simulink model "HeliDraft_06_02_2025_13_24pm"  (R2024b)
settings: Solver=VariableStepAuto  StartTime=0.0  StopTime=10.0  RelTol=1e-3
undefined symbols (not defined in the file or in its folder): AngVel, AngVeltr, Earth, MTOW, WGS84
libraries: aerolibatmos2 x2, aerolibanimutils x2, aerolibfltsims x2, aerolibtransform2 x1, shared6dof x1
settings Model: Creator=stand-alone1  LastModifiedBy=stand-alone1

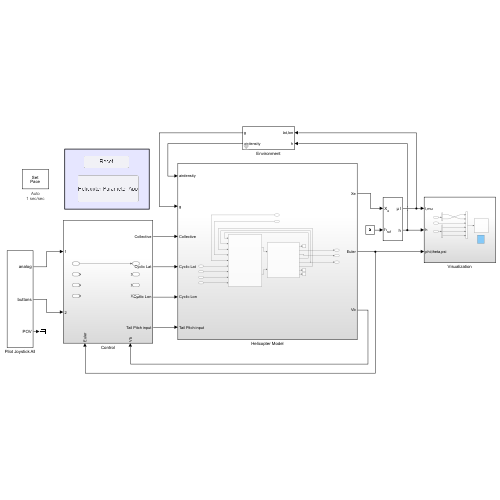
[thumbnail: Simulink's stored preview of the top-level diagram]
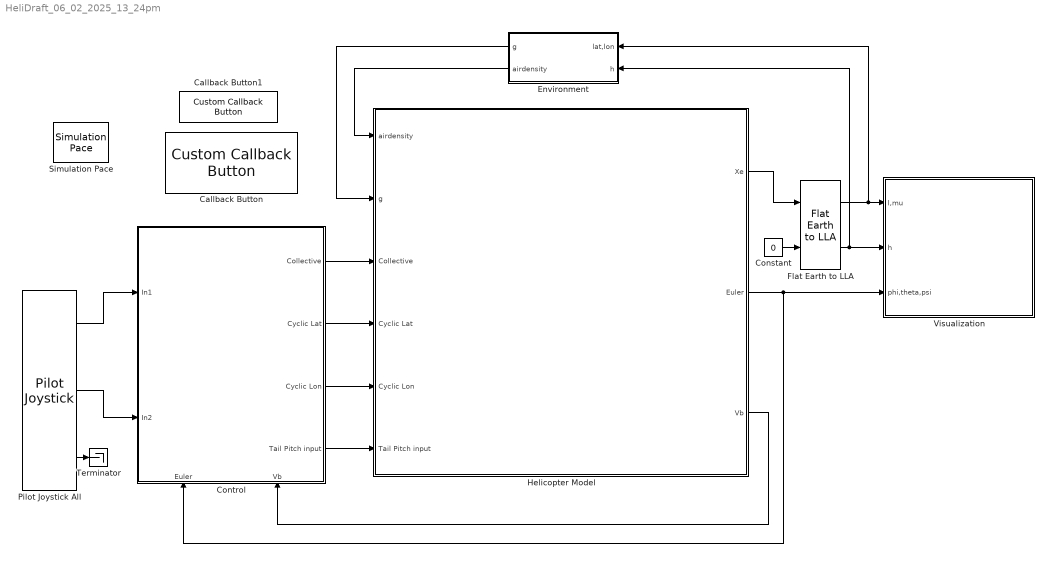
== system HeliDraft_06_02_2025_13_24pm ==
  Callback Button : CustomCallbackButton  Configuration="{\"components\":[{\"name\":\"BackgroundImageComponent\",\"settings\":{\"image\":{\"size\":[0,0],\"src\":\"default\",\"srcOrientation\":\"Right\"},\"position\":[0,0,1,1]}},{\"name\":\"ButtonStateComponent\",\"settings\":{\"buttonType\":\"momentary\",\"clickFcn\":\"run(\\\"HelicopterParameterEstimation.mlapp\\\");\",\"onValue\":1,\"position\":[0,0,1,1],\"pressDelay\":\"500\",\"pressFcn\":\"\",\"repeatInterval\":\"0\",\"states\":[{\"horizontalAlignment\":\"center\",\"image\":{\"position\":[0,0,1,1],\"size\":[1,1],\"src\":\"default\",\"srcOrientation\":\"Right\"},\"label\":{\"color\":[0.01176470588,0.01176470588,0.01176470588,1],\"icon\":{\"size\":[0,0],\"src\":\"default\",\"srcOrientation\":\"Right\"},\"iconOffset\":0,\"iconPlacement\":\"left\",\"opacity\":1,\"show\":true,\"text\":{\"content\":\"Helicopter Parameter App\",\"font\":\"Helvetica\"}},\"labelOffset\":[0,0],\"verticalAlignment\":\"middle\"},{\"horizontalAlignment\":\"center\",\"image\":{\"position\":[0,0,1,1],\"size\":[1,1],\"src\":\"default\",\"srcOrientation\":\"Right\"},\"label\":{\"color\":[0.01176470588,0.01176470588,0.01176470588,1],\"icon\":{\"size\":[0,0],\"src\":\"default\",\"srcOrientation\":\"Right\"},\"iconOffset\":0,\"iconPlacement\":\"left\",\"opacity\":1,\"show\":true,\"text\":{\"content\":\"Helicopter Parameter App\",\"font\":\"Helvetica\"}},\"labelOffset\":[0,0],\"verticalAlignment\":\"middle\"},{\"horizontalAlignment\":\"center\",\"image\":{\"position\":[0,0,1,1],\"size\":[1,1],\"src\":\"default\",\"srcOrientation\":\"Right\"},\"label\":{\"color\":[0.01176470588,0.01176470588,0.01176470588,1],\"icon\":{\"size\":[0,0],\"src\":\"default\",\"srcOrientation\":\"Right\"},\"iconOffset\":0,\"iconPlacement\":\"left\",\"opacity\":1,\"show\":true,\"text\":{\"content\":\"Helicopter Parameter App\",\"font\":\"Helvetica\"}},\"labelOffset\":[0,0],\"verticalAlignment\":\"middle\"},{\"horizontalAlignment\":\"center\",\"image\":{\"position\":[0,0,1,1],\"size\":[1,1],\"src\":\"default\",\"srcOrientation\":\"Right\"},\"label\":{\"color\":[0.01176470588,0.01176470588,0.01176470588,1],\"icon\":{\"size\":[0,0],\"src\":\"default\",\"srcOrientation\":\"Right\"},\"iconOffset\":0,\"iconPlacement\":\"left\",\"opacity\":1,\"show\":true,\"text\":{\"content\":\"Helicopter Parameter App\",\"font\":\"Helvetica\"}},\"labelOffset\":[0,0],\"verticalAlignment\":\"middle\"}]}},{\"name\":\"ForegroundImageComponent\",\"settings\":{\"image\":{\"size\":[0,0],\"src\":\"default\",\"srcOrientation\":\"Right\"},\"isForeground\":1,\"position\":[0,0,1,1]}}],\"settings\":{\"BindingType\":\"standalone\",\"backgroundColor\":[244,244,244,1],\"backgroundOffset\":0.2,\"backgroundOpacity\":1,\"fixedAspectRatio\":\"off\",\"foregroundColor\":[0.01176470588,0.01176470588,0.01176470588,1],\"migratedFromLegacy\":true,\"useBackgroundColor\":true,\"variant\":\"callback\",\"version\":\"R2023a\"},\"type\":\"Button\"}"  CustomBackgroundColor="{\"color\":[0.9568627451,0.9568627451,0.9568627451],\"show\":true}"
  Callback Button1 : CustomCallbackButton  Configuration="{\"components\":[{\"name\":\"BackgroundImageComponent\",\"settings\":{\"image\":{\"size\":[0,0],\"src\":\"default\",\"srcOrientation\":\"Right\"},\"position\":[0,0,1,1]}},{\"name\":\"ButtonStateComponent\",\"settings\":{\"buttonType\":\"momentary\",\"clickFcn\":\"clc; clear; close all;\",\"onValue\":1,\"position\":[0,0,1,1],\"pressDelay\":\"500\",\"pressFcn\":\"\",\"repeatInterval\":\"0\",\"states\":[{\"horizontalAlignment\":\"center\",\"image\":{\"position\":[0,0,1,1],\"size\":[1,1],\"src\":\"default\",\"srcOrientation\":\"Right\"},\"label\":{\"color\":[0.01176470588,0.01176470588,0.01176470588,1],\"icon\":{\"size\":[0,0],\"src\":\"default\",\"srcOrientation\":\"Right\"},\"iconOffset\":0,\"iconPlacement\":\"left\",\"opacity\":1,\"show\":true,\"text\":{\"content\":\"Reset\",\"font\":\"Helvetica\"}},\"labelOffset\":[0,0],\"verticalAlignment\":\"middle\"},{\"horizontalAlignment\":\"center\",\"image\":{\"position\":[0,0,1,1],\"size\":[1,1],\"src\":\"default\",\"srcOrientation\":\"Right\"},\"label\":{\"color\":[0.01176470588,0.01176470588,0.01176470588,1],\"icon\":{\"size\":[0,0],\"src\":\"default\",\"srcOrientation\":\"Right\"},\"iconOffset\":0,\"iconPlacement\":\"left\",\"opacity\":1,\"show\":true,\"text\":{\"content\":\"Reset\",\"font\":\"Helvetica\"}},\"labelOffset\":[0,0],\"verticalAlignment\":\"middle\"},{\"horizontalAlignment\":\"center\",\"image\":{\"position\":[0,0,1,1],\"size\":[1,1],\"src\":\"default\",\"srcOrientation\":\"Right\"},\"label\":{\"color\":[0.01176470588,0.01176470588,0.01176470588,1],\"icon\":{\"size\":[0,0],\"src\":\"default\",\"srcOrientation\":\"Right\"},\"iconOffset\":0,\"iconPlacement\":\"left\",\"opacity\":1,\"show\":true,\"text\":{\"content\":\"Reset\",\"font\":\"Helvetica\"}},\"labelOffset\":[0,0],\"verticalAlignment\":\"middle\"},{\"horizontalAlignment\":\"center\",\"image\":{\"position\":[0,0,1,1],\"size\":[1,1],\"src\":\"default\",\"srcOrientation\":\"Right\"},\"label\":{\"color\":[0.01176470588,0.01176470588,0.01176470588,1],\"icon\":{\"size\":[0,0],\"src\":\"default\",\"srcOrientation\":\"Right\"},\"iconOffset\":0,\"iconPlacement\":\"left\",\"opacity\":1,\"show\":true,\"text\":{\"content\":\"Reset\",\"font\":\"Helvetica\"}},\"labelOffset\":[0,0],\"verticalAlignment\":\"middle\"}]}},{\"name\":\"ForegroundImageComponent\",\"settings\":{\"image\":{\"size\":[0,0],\"src\":\"default\",\"srcOrientation\":\"Right\"},\"isForeground\":1,\"position\":[0,0,1,1]}}],\"settings\":{\"BindingType\":\"standalone\",\"backgroundColor\":[244,244,244,1],\"backgroundOffset\":0.2,\"backgroundOpacity\":1,\"fixedAspectRatio\":\"off\",\"foregroundColor\":[0.01176470588,0.01176470588,0.01176470588,1],\"migratedFromLegacy\":true,\"useBackgroundColor\":true,\"variant\":\"callback\",\"version\":\"R2023a\"},\"type\":\"Button\"}"  CustomBackgroundColor="{\"color\":[0.9568627451,0.9568627451,0.9568627451],\"show\":true}"
  Constant : Constant  Value=0
  Control : Subsystem
      settings: PortSchema="{\"entries\":[{\"content\":{\"sides\":[{\"content\":{\"connectorIds\":[\"In1\",\"In2\"]},\"type\":\"ConnectorPlacement.EquallySpacedRectSide\",\"uuid\":\"528401e7-0fef-44be-ba63-acf96d247fb7\"},{\"content\":{\"connectorIds\":[\"Out1\",\"Out2\",\"Out3\",\"Out4\"],\"side\":\"RIGHT\"},\"type\":\"ConnectorPlacement.EquallySpacedRectSide\",\"uuid\":\"314663aa-6cd9-4175-a49a-1575f8a7b87b\"},{\"content\":{\"side\":\"TOP\"},\"type\":\"ConnectorPlacement.EquallySpacedRectSide\",\"uuid\":\"d6c3b2b9-365b-49fe-86cc-8f0c15878230\"},{\"content\":{\"connectorIds\":[\"In3\",\"In4\"],\"side\":\"BOTTOM\"},\"type\":\"ConnectorPlacement.EquallySpacedRectSide\",\"uuid\":\"be77d0ba-d3ca-47ac-ab5e-0cf95d8527f7\"}]},\"type\":\"ConnectorPlacement.EquallySpacedConnector\",\"uuid\":\"719848b2-01be-4853-b472-0e21e9b8be5c\"}],\"packageUris\":[\"http://schema.mathworks.com/mf0/Connector/R2020b\"],\"version\":\"1.0\"}"
  Environment : Subsystem  mask{consg=on, atmomodel=ISA}
      mask prompts: consg "Constant g (Gravitational Acceleration)"; atmomodel "Atmosphere Model"
      mask DialogControl a Prompt: Environment
      mask DialogControl b Prompt: Atmosphere properties and gravity model
      mask DialogControl c Prompt: Decisions
  Flat Earth to LLA : aerolibtransform2/Flat Earth to LLA  units=Metric (MKS)  ptype=Earth (WGS84)  F=1/298.257223563  R=6378137  refPosPort=off  LL0=[0 10]  psi=0
  Helicopter Model : Subsystem
  Pilot Joystick All : aerolibanimutils/Pilot Joystick  JoystickID=Joystick1  OutputConfiguration=AllOutputs  SampleTime=1/30
      settings: LibrarySourceBlock=aerolibanimutils/Pilot Joystick All
  Simulation Pace : aerolibanimutils/Simulation Pace  SimulationPace=1  SleepMode=Auto  OutputPaceError=off  SampleTime=1/30
  Terminator : Terminator
  Visualization : Subsystem
  wires:
  Constant/1 -> Flat Earth to LLA/2
  Flat Earth to LLA/1 -> Visualization/1(l,mu), Environment/1(lat,lon)
  Flat Earth to LLA/2 -> Visualization/2(h), Environment/2(h)
  Pilot Joystick All/1 -> Control/1(In1)
  Pilot Joystick All/2 -> Control/2(In2)
  Environment/1(g) -> Helicopter Model/2(g)
  Environment/2(airdensity) -> Helicopter Model/1(airdensity)
  Helicopter Model/1(Xe) -> Flat Earth to LLA/1
  Helicopter Model/2(Euler) -> Visualization/3(phi,theta,psi), Control/3(Euler)
  Control/1(Collective) -> Helicopter Model/3(Collective)
  Control/2(Cyclic Lat) -> Helicopter Model/4(Cyclic Lat)
  Control/3(Cyclic Lon) -> Helicopter Model/5(Cyclic Lon)
  Control/4(Tail Pitch input) -> Helicopter Model/6(Tail Pitch input)
  Pilot Joystick All/3 -> Terminator/1
  Helicopter Model/3(Vb) -> Control/4(Vb)

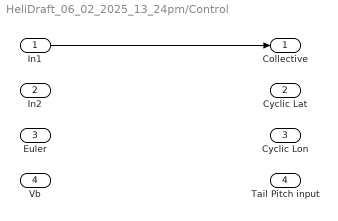
== system HeliDraft_06_02_2025_13_24pm/Control ==
  In1 : Inport
  In2 : Inport  Port=2
  Euler : Inport  Port=3
  Vb : Inport  Port=4
  Collective : Outport
  Cyclic Lat : Outport  Port=2
  Cyclic Lon : Outport  Port=3
  Tail Pitch input : Outport  Port=4
  wires:
  In1/1 -> Collective/1

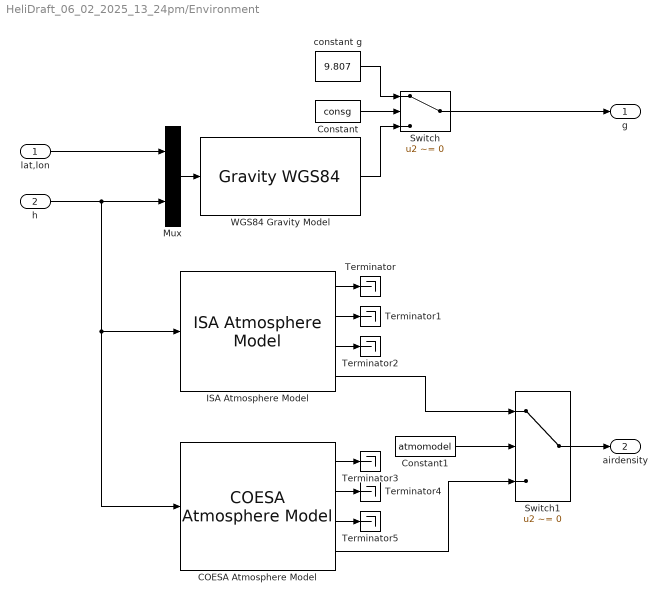
== system HeliDraft_06_02_2025_13_24pm/Environment ==
  lat,lon : Inport
  h : Inport  Port=2
  COESA Atmosphere Model : aerolibatmos2/COESA Atmosphere Model  units=Metric (MKS)  spec=1976 COESA-extended U.S. Standard Atmosphere  model=Profile  profile_var=High temperature  profile_percent=1%  profile_alt=5 km (16404 ft)  envelope_var=High temperature  envelope_percent=1%  action=Warning
  Constant : Constant  Value=consg
  Constant1 : Constant  Value=atmomodel
  ISA Atmosphere Model : aerolibatmos2/ISA Atmosphere Model  useExtended=off  action=Warning  custom=off  viscosityOut=off  g=9.80665  gamma=1.4  R=287.0531  L=0.0065  h_trop=11000  h_strat=20000  rho0=1.225  P0=101325  T0=288.15  h0=0  S=110.4  Tref=273.15  muref=1.716e-5
  Mux : Mux  Inputs=2
  Switch : Switch  Criteria=u2 ~= 0  SaturateOnIntegerOverflow=off  InputSameDT=off
  Switch1 : Switch  Criteria=u2 ~= 0  SaturateOnIntegerOverflow=off  InputSameDT=off
  Terminator{,1..5} (6 alike) : Terminator
  "WGS84 Gravity Model  " : GravityWGS84
  constant g : Constant  Value=9.807
  g : Outport
  airdensity : Outport  Port=2
  wires:
  lat,lon/1 -> Mux/1
  Constant/1 -> Switch/2
  constant g/1 -> Switch/1
  "WGS84 Gravity Model  "/1 -> Switch/3
  Switch/1 -> g/1
  Mux/1 -> "WGS84 Gravity Model  "/1
  h/1 -> COESA Atmosphere Model/1, ISA Atmosphere Model/1, Mux/2
  Switch1/1 -> airdensity/1
  ISA Atmosphere Model/1 -> Terminator/1
  ISA Atmosphere Model/2 -> Terminator1/1
  ISA Atmosphere Model/3 -> Terminator2/1
  COESA Atmosphere Model/2 -> Terminator4/1
  COESA Atmosphere Model/1 -> Terminator3/1
  COESA Atmosphere Model/3 -> Terminator5/1
  ISA Atmosphere Model/4 -> Switch1/1
  COESA Atmosphere Model/4 -> Switch1/3
  Constant1/1 -> Switch1/2

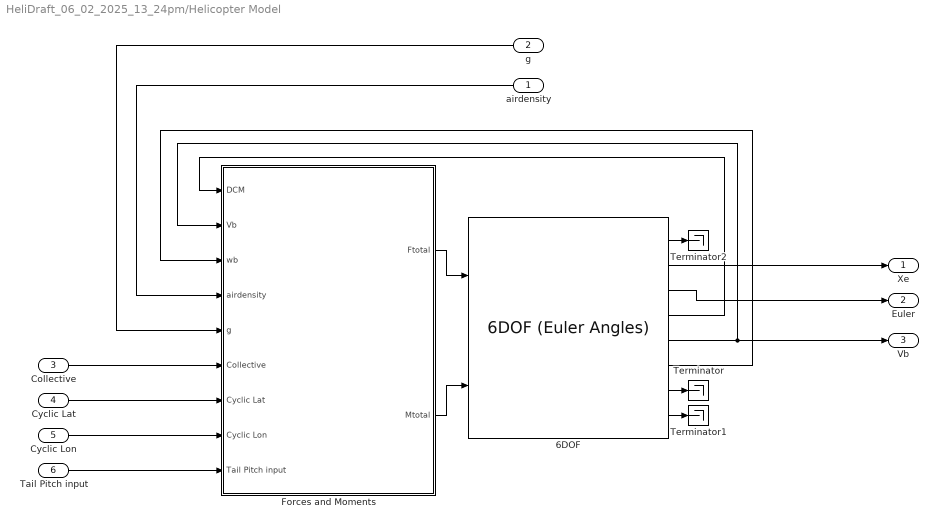
== system HeliDraft_06_02_2025_13_24pm/Helicopter Model ==
  airdensity : Inport
  g : Inport  Port=2
  Collective : Inport  Port=3
  Cyclic Lat : Inport  Port=4
  Cyclic Lon : Inport  Port=5
  Tail Pitch input : Inport  Port=6
  6DOF : shared6dof/6DOF (Euler Angles)  units=Metric (MKS)  mtype=Fixed  rep=Euler Angles  xme_0=[0 0 0]  Vm_0=[0 0 0]  eul_0=[0 0 0]  pm_0=[0 0 0]  mass_0=MTOW  mass_e=0.5  mass_f=2.0  inertia=eye(3)  inertia_e=eye(3)  inertia_f=2*eye(3)  k_quat=1.0  vre_flag=off  abi_flag=off  aMode=0  xme_statename=''  Vm_statename=''  eul_statename=''  quat_statename=''  pm_statename=''  mass_statename=''
  Forces and Moments : Subsystem
  Terminator : Terminator
  Terminator1 : Terminator
  Terminator2 : Terminator
  Xe : Outport
  Euler : Outport  Port=2
  Vb : Outport  Port=3
  wires:
  6DOF/1 -> Terminator2/1
  6DOF/8 -> Terminator1/1
  Forces and Moments/1(Ftotal) -> 6DOF/1
  Forces and Moments/2(Mtotal) -> 6DOF/2
  6DOF/6 -> Forces and Moments/3(wb)
  6DOF/4 -> Forces and Moments/1(DCM)
  6DOF/7 -> Terminator/1
  6DOF/5 -> Vb/1, Forces and Moments/2(Vb)
  Cyclic Lat/1 -> Forces and Moments/7(Cyclic Lat)
  Collective/1 -> Forces and Moments/6(Collective)
  6DOF/3 -> Euler/1
  Tail Pitch input/1 -> Forces and Moments/9(Tail Pitch input)
  Cyclic Lon/1 -> Forces and Moments/8(Cyclic Lon)
  airdensity/1 -> Forces and Moments/4(airdensity)
  g/1 -> Forces and Moments/5(g)
  6DOF/2 -> Xe/1

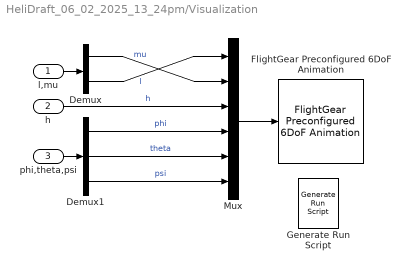
== system HeliDraft_06_02_2025_13_24pm/Visualization ==
  l,mu : Inport
  h : Inport  Port=2
  phi,theta,psi : Inport  Port=3
  Demux : Demux  Outputs=2
  Demux1 : Demux  Outputs=3
  "FlightGear Preconfigured 6DoF Animation " : aerolibfltsims/FlightGear Preconfigured 6DoF Animation  xFlightGearVersion=v2019.1  DestinationIpAddress=127.0.0.1  DestinationPort=5502  SampleTime=1/30  packetVersion=24
  "Generate Run Script " : aerolibfltsims/Generate Run Script  Architecture=Default  dataFlow=Send  GeometryModelName=HL20  AirportId=KSFO  RunwayId=10L  InitialAltitude=7224  InitialHeading=113  OffsetDistance=4.72  OffsetAzimuth=0  InstallScenery=off  DisableShaders=off  OriginAddress=127.0.0.1  DestinationPort=5502  OriginPort=5505  LocalAddress=127.0.0.1  OutputFileName=runfg.bat  FlightGearBaseDirectory=C:\Program Files\FlightGear
  Mux : Mux  Inputs=6
  wires:
  l,mu/1 -> Demux/1
  Demux/2 -> Mux/1  "l"
  Demux/1 -> Mux/2  "mu"
  Mux/1 -> "FlightGear Preconfigured 6DoF Animation "/1
  h/1 -> Mux/3  "h"
  Demux1/1 -> Mux/4  "phi"
  Demux1/2 -> Mux/5  "theta"
  Demux1/3 -> Mux/6  "psi"
  phi,theta,psi/1 -> Demux1/1

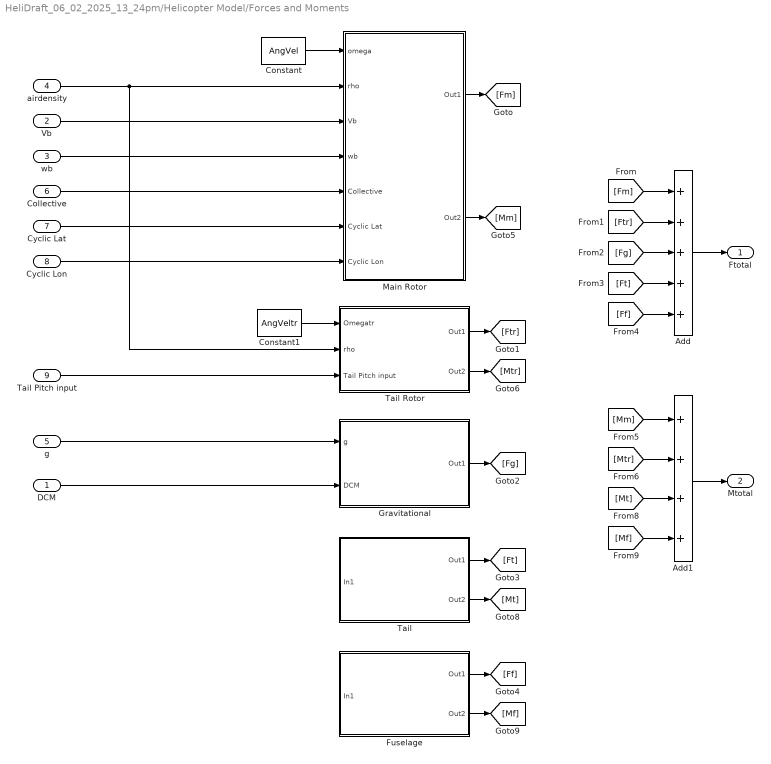
== system HeliDraft_06_02_2025_13_24pm/Helicopter Model/Forces and Moments ==
  DCM : Inport
  Vb : Inport  Port=2
  wb : Inport  Port=3
  airdensity : Inport  Port=4
  g : Inport  Port=5
  Collective : Inport  Port=6
  Cyclic Lat : Inport  Port=7
  Cyclic Lon : Inport  Port=8
  Tail Pitch input : Inport  Port=9
  Add : Sum  Inputs=+++++
  Add1 : Sum  Inputs=++++
  Constant : Constant  Value=AngVel
  Constant1 : Constant  Value=AngVeltr
  Fuselage : Subsystem
  Gravitational : Subsystem
  Main Rotor : Subsystem
  Tail : Subsystem
  Tail Rotor : Subsystem
  Ftotal : Outport
  Mtotal : Outport  Port=2
  wires:
  Add/1 -> Ftotal/1
  Add1/1 -> Mtotal/1
  Main Rotor/1(Out1) -> [Fm]
  Tail Rotor/1(Out1) -> [Ftr]
  Gravitational/1(Out1) -> [Fg]
  Tail/1(Out1) -> [Ft]
  Fuselage/1(Out1) -> [Ff]
  [Fm] -> Add/1
  [Ftr] -> Add/2
  [Fg] -> Add/3
  [Ft] -> Add/4
  [Ff] -> Add/5
  Main Rotor/2(Out2) -> [Mm]
  Tail Rotor/2(Out2) -> [Mtr]
  Tail/2(Out2) -> [Mt]
  Fuselage/2(Out2) -> [Mf]
  [Mm] -> Add1/1
  [Mtr] -> Add1/2
  [Mf] -> Add1/4
  [Mt] -> Add1/3
  Constant/1 -> Main Rotor/1(omega)
  Constant1/1 -> Tail Rotor/1(Omegatr)
  airdensity/1 -> Tail Rotor/2(rho), Main Rotor/2(rho)
  g/1 -> Gravitational/1(g)
  DCM/1 -> Gravitational/2(DCM)
  Collective/1 -> Main Rotor/5(Collective)
  Tail Pitch input/1 -> Tail Rotor/3(Tail Pitch input)
  Cyclic Lat/1 -> Main Rotor/6(Cyclic Lat)
  Cyclic Lon/1 -> Main Rotor/7(Cyclic Lon)
  wb/1 -> Main Rotor/4(wb)
  Vb/1 -> Main Rotor/3(Vb)

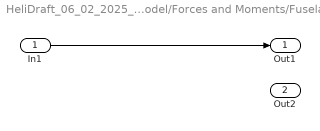
== system HeliDraft_06_02_2025_13_24pm/Helicopter Model/Forces and Moments/Fuselage ==
  In1 : Inport
  Out1 : Outport
  Out2 : Outport  Port=2
  wires:
  In1/1 -> Out1/1

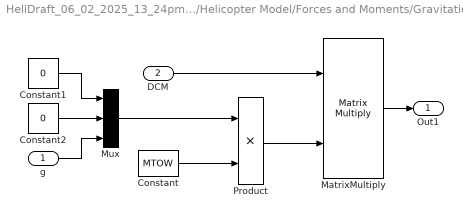
== system HeliDraft_06_02_2025_13_24pm/Helicopter Model/Forces and Moments/Gravitational ==
  g : Inport
  DCM : Inport  Port=2
  Constant : Constant  Value=MTOW
  Constant1 : Constant  Value=0
  Constant2 : Constant  Value=0
  MatrixMultiply : Product  Multiplication=Matrix(*)
  Mux : Mux  Inputs=3
  Product : Product
  Out1 : Outport
  wires:
  DCM/1 -> MatrixMultiply/1
  MatrixMultiply/1 -> Out1/1
  Product/1 -> MatrixMultiply/2
  g/1 -> Mux/3
  Constant/1 -> Product/2
  Mux/1 -> Product/1
  Constant1/1 -> Mux/1
  Constant2/1 -> Mux/2

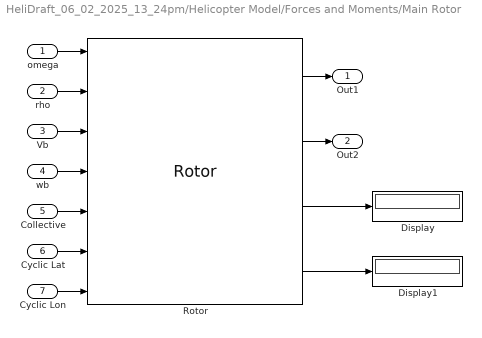
== system HeliDraft_06_02_2025_13_24pm/Helicopter Model/Forces and Moments/Main Rotor ==
  omega : Inport
  rho : Inport  Port=2
  Vb : Inport  Port=3
  wb : Inport  Port=4
  Collective : Inport  Port=5
  Cyclic Lat : Inport  Port=6
  Cyclic Lon : Inport  Port=7
  Display : Display
  Display1 : Display
  Rotor : Rotor  modelMode=With flap effects  controlInput=on  CTCQMode=Compute using BEMT  Nb=Nb  CTout=on  radius=R  chord=c
  Out1 : Outport
  Out2 : Outport  Port=2
  wires:
  omega/1 -> Rotor/1
  Rotor/1 -> Out1/1
  rho/1 -> Rotor/2
  Rotor/2 -> Out2/1
  Collective/1 -> Rotor/5
  Rotor/3 -> Display/1
  Rotor/4 -> Display1/1
  Cyclic Lon/1 -> Rotor/7
  Cyclic Lat/1 -> Rotor/6
  Vb/1 -> Rotor/3
  wb/1 -> Rotor/4

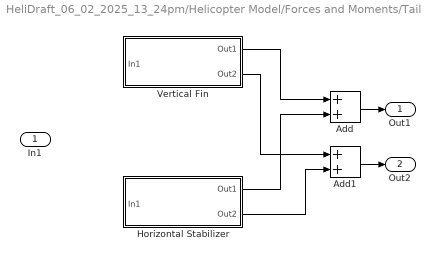
== system HeliDraft_06_02_2025_13_24pm/Helicopter Model/Forces and Moments/Tail ==
  In1 : Inport
  Add : Sum
  Add1 : Sum
  Horizontal Stabilizer : Subsystem
  Vertical Fin : Subsystem
  Out1 : Outport
  Out2 : Outport  Port=2
  wires:
  Vertical Fin/1(Out1) -> Add/1
  Horizontal Stabilizer/1(Out1) -> Add/2
  Add/1 -> Out1/1
  Add1/1 -> Out2/1
  Horizontal Stabilizer/2(Out2) -> Add1/2
  Vertical Fin/2(Out2) -> Add1/1

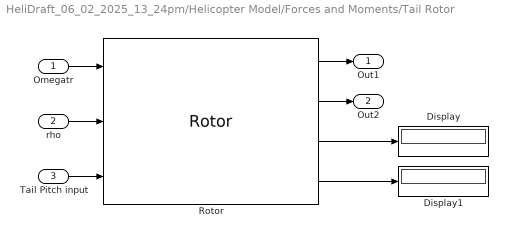
== system HeliDraft_06_02_2025_13_24pm/Helicopter Model/Forces and Moments/Tail Rotor ==
  Omegatr : Inport
  rho : Inport  Port=2
  Tail Pitch input : Inport  Port=3
  Display : Display
  Display1 : Display
  Rotor : Rotor  controlInput=on  CTCQMode=Compute using BEMT  Nb=Nbtr  CTout=on  radius=Rtr
  Out1 : Outport
  Out2 : Outport  Port=2
  wires:
  Omegatr/1 -> Rotor/1
  rho/1 -> Rotor/2
  Rotor/2 -> Out2/1
  Rotor/1 -> Out1/1
  Rotor/3 -> Display/1
  Rotor/4 -> Display1/1
  Tail Pitch input/1 -> Rotor/3

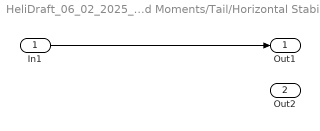
== system HeliDraft_06_02_2025_13_24pm/Helicopter Model/Forces and Moments/Tail/Horizontal Stabilizer ==
  In1 : Inport
  Out1 : Outport
  Out2 : Outport  Port=2
  wires:
  In1/1 -> Out1/1

== system HeliDraft_06_02_2025_13_24pm/Helicopter Model/Forces and Moments/Tail/Vertical Fin ==
  In1 : Inport
  Out1 : Outport
  Out2 : Outport  Port=2
  wires:
  In1/1 -> Out1/1
